simulink model "StateObserverTest3"  (R2018b)
settings: Solver=VariableStepAuto  StartTime=0.0  StopTime=30  RelTol=1e-3
values from neighbouring files (symbols this model uses):
  GdSpeed = c2d(Gspeed,Ts,'tustin')    [DiscreteObserverAndSFB.m]
  K = -lqrd (Aaugmented,Baugmented,Qespeed,Respeed,Ts)    [DiscreteObserverAndSFB.m]
  Ltr = L'    [DiscreteObserverAndSFB.m]
  Ts = 0.01    [DiscreteObserverAndSFB.m]
undefined symbols (not defined in the file or in its folder): DiscIntNeverNeededParam
settings Model: Creator=mmbio  LastModifiedBy=Yahya

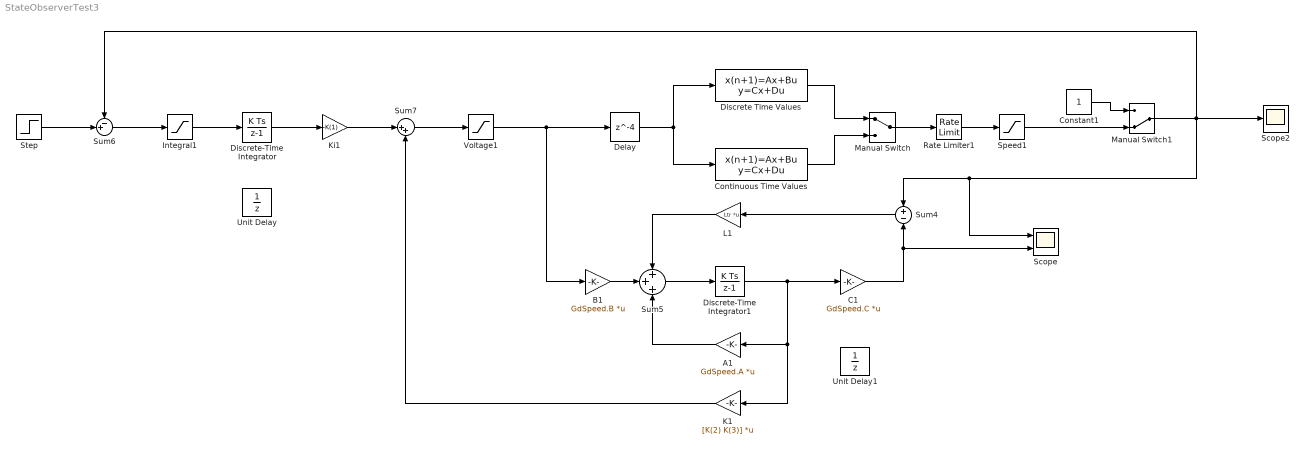
== system StateObserverTest3 ==
  A1 : Gain  Gain=GdSpeed.A  Multiplication=Matrix(K*u)
  B1 : Gain  Gain=GdSpeed.B  Multiplication=Matrix(K*u)
  C1 : Gain  Gain=GdSpeed.C  Multiplication=Matrix(K*u)
  Constant1 : Constant
  Continuous Time Values : DiscreteStateSpace  A=[-1.14 -1.36; 1 0]  B=[1; 0]  C=[0 1.507]  D=0  SampleTime=0.01
  Delay : Delay  DelayLength=4  SampleTime=Ts
  Discrete Time Values : DiscreteStateSpace  A=GdSpeed.A  B=GdSpeed.B  C=GdSpeed.C  D=0  SampleTime=Ts
  Discrete-Time Integrator : DiscreteIntegrator  SampleTime=Ts  ICPrevOutput=DiscIntNeverNeededParam  ICPrevScaledInput=DiscIntNeverNeededParam
  Discrete-Time Integrator1 : DiscreteIntegrator  SampleTime=Ts  ICPrevOutput=DiscIntNeverNeededParam  ICPrevScaledInput=DiscIntNeverNeededParam
  Integral1 : Saturate  UpperLimit=5/0.5  LowerLimit=-5/0.5
  K1 : Gain  Gain=[K(2) K(3)]  Multiplication=Matrix(K*u)
  Ki1 : Gain  Gain=-K(1)
  L1 : Gain  Gain=Ltr  Multiplication=Matrix(K*u)
  Manual Switch : ManualSwitch
  Manual Switch1 : ManualSwitch  CurrentSetting=0
  Rate Limiter1 : RateLimiter  RisingSlewLimit=0.65  FallingSlewLimit=-0.65  SampleTimeMode=inherited
  Scope : Scope  NumInputPorts=2
  Scope2 : Scope
  Speed1 : Saturate  UpperLimit=1000  LowerLimit=0
  Step : Step  SampleTime=0
  Sum4 : Sum  Inputs=+-
  Sum5 : Sum  Inputs=+++
  Sum6 : Sum  Inputs=-+|
  Sum7 : Sum  Inputs=|++
  Unit Delay : UnitDelay  SampleTime=Ts
  Unit Delay1 : UnitDelay  SampleTime=Ts
  Voltage1 : Saturate  UpperLimit=5  LowerLimit=0
  wires:
  Speed1/1 -> Manual Switch1/2
  A1/1 -> Sum5/3
  Sum4/1 -> L1/1
  Constant1/1 -> Manual Switch1/1
  Discrete-Time Integrator1/1 -> C1/1, K1/1, A1/1
  B1/1 -> Sum5/2
  Discrete-Time Integrator/1 -> Ki1/1
  Rate Limiter1/1 -> Speed1/1
  L1/1 -> Sum5/1
  Sum7/1 -> Voltage1/1
  Voltage1/1 -> Delay/1, B1/1
  Sum5/1 -> Discrete-Time Integrator1/1
  Step/1 -> Sum6/2
  C1/1 -> Scope/2, Sum4/2
  Sum6/1 -> Integral1/1
  Integral1/1 -> Discrete-Time Integrator/1
  K1/1 -> Sum7/2
  Manual Switch1/1 -> Scope/1, Sum4/1, Scope2/1, Sum6/1
  Ki1/1 -> Sum7/1
  Delay/1 -> Discrete Time Values/1, Continuous Time Values/1
  Manual Switch/1 -> Rate Limiter1/1
  Discrete Time Values/1 -> Manual Switch/1
  Continuous Time Values/1 -> Manual Switch/2
